simulink model "backstepping_last_good"  (R2023a)
settings: Solver=ode23t  StartTime=0.0  StopTime=inf  RelTol=1e-3
undefined symbols (not defined in the file): K1, K10, K11, K12, K2, K3, K4, K5, K6, K7, K8, K9
libraries: simulink x1, vrlib x1
settings Model: Creator=sait karadeniz  LastModifiedBy=sait karadeniz
settings DataIOCC: ReturnWorkspaceOutputs=off

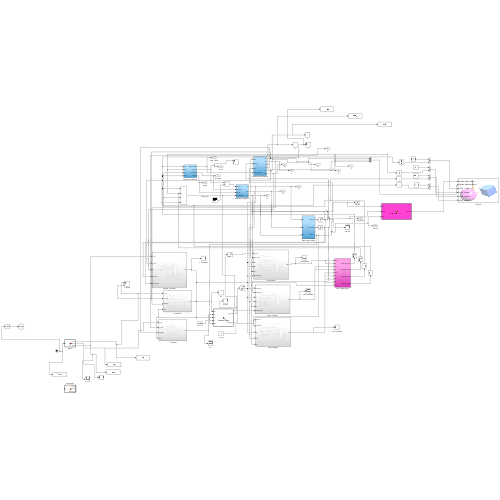
[thumbnail: Simulink's stored preview of the top-level diagram]
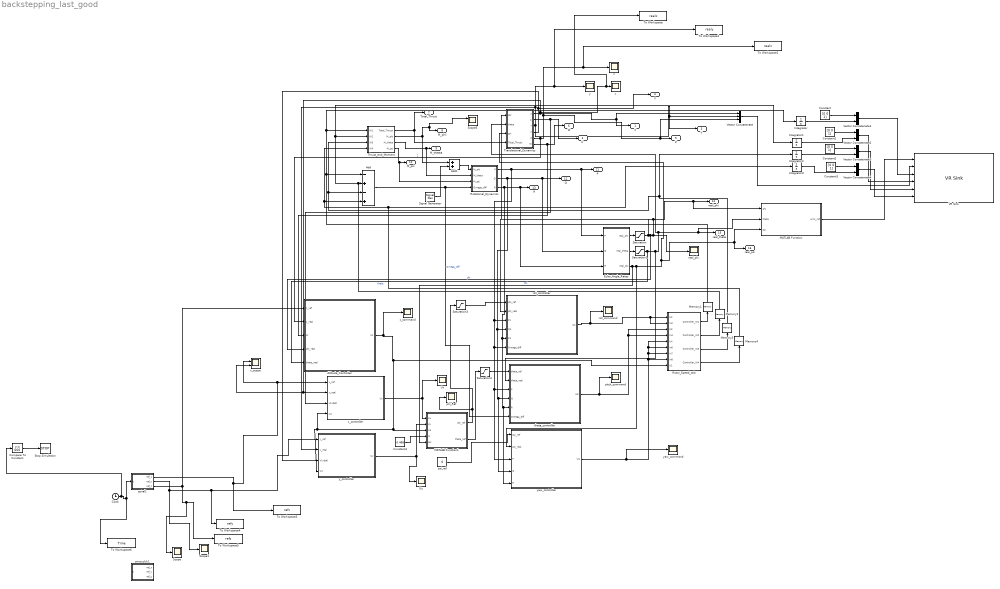
== system backstepping_last_good ==
  Add : Sum  Inputs=-+-+
  Add1 : Sum
  Altitude_Controller : Subsystem
  Clock : Clock
  Compare To Constant : simulink/Logic and Bit Operations/Compare To Constant  relop=>=  const=600  OutDataTypeStr=boolean
  Constant{,1..3} (4 alike) : Constant  Value=[0 0 1]  OutMax=[3]
  Constant4 : Constant  Value=0.468
  Euler_Angle_Rates : Subsystem
  Integrator{,1..3} (4 alike) : Integrator
  MATLAB Function : MATLAB Function  TreatAsAtomicUnit=on
  MATLAB Function1 : MATLAB Function  TreatAsAtomicUnit=on
  Memory{1..4} (4 alike) : Memory
  Rotational_Dynamics : Subsystem
  Rotor_Speed_calc : Subsystem
  Saturation : Saturate  UpperLimit=pi/2  LowerLimit=-pi/2
  Saturation1 : Saturate  UpperLimit=pi/2  LowerLimit=-pi/2
  Saturation2 : Saturate  UpperLimit=0.3  LowerLimit=-0.3
  Saturation3 : Saturate  UpperLimit=0.3  LowerLimit=-0.3
  Scope : Scope
  Scope1 : Scope
  Scope5 : Scope  NumInputPorts=2
  Signal Generator : SignalGenerator  Amplitude=0  Frequency=2  Units=rad/sec
  Stop Simulation : Stop
  Thrust_and_Moment : Subsystem
  To Workspace : ToWorkspace  VariableName=realx  SampleTime=-1
  To Workspace1 : ToWorkspace  VariableName=realy  SampleTime=-1
  To Workspace2 : ToWorkspace  VariableName=realz  SampleTime=-1
  To Workspace3 : ToWorkspace  VariableName=refx  SampleTime=-1
  To Workspace4 : ToWorkspace  VariableName=refy  SampleTime=-1
  To Workspace5 : ToWorkspace  VariableName=refz  SampleTime=-1
  To Workspace6 : ToWorkspace  VariableName=Time  SampleTime=-1
  Translational_Dynamics : Subsystem
  Ux : Scope
  Uy : Scope
  VR Sink : vrlib/VR Sink  InstantiateOnLoad=on  SampleTime=0.1  ViewEnable=on  RemoteChange=off  RemoteView=off  FieldsWritten=DRONE_BODY.rotation.4.1.1.double#DRONE_BODY.translation.3.1.1.double#PROP_1.rotation.4.1.1.double#PROP_2.rotation.4.1.1.double#PROP_3.rotation.4.1.1.double#PROP_4.rotation.4.1.1.double  WorldFileName=C:\Documents\quadcopter.wrl  WorldDescription=Quadcopter World  AutoView=on  VideoDimensions=[]  AllowVariableSize=off
  Vector Concatenate : Concatenate  NumInputs=3
  Vector Concatenate{1..4} (4 alike) : Concatenate
  phi_Ref : Scope
  pitch_command : Scope
  psi_ref : Constant  Value=0
  real_phi. : Scope
  roll_command : Scope
  roll_controller : Subsystem
  sonsuzluk1 : MATLAB Function  TreatAsAtomicUnit=on
  spiral1 : MATLAB Function  TreatAsAtomicUnit=on
  theta_controller : Subsystem
  x : Scope
  x_controller : Subsystem
  x_scope : Scope  NumInputPorts=2
  y : Scope
  y_controller : Subsystem
  yaw_command : Scope
  yaw_controller : Subsystem
  z : Scope
  z_command : Scope
  X : Outport
  U : Outport  Port=2
  Y : Outport  Port=3
  V : Outport  Port=4
  Z : Outport  Port=5
  W : Outport  Port=6
  Total_Thrust : Outport  Port=7
  M_phii : Outport  Port=8
  M_thetaa : Outport  Port=9
  M_psi : Outport  Port=10
  P : Outport  Port=11
  Q : Outport  Port=12
  R : Outport  Port=13
  real_phi : Outport  Port=14
  real_theta : Outport  Port=15
  real_psi : Outport  Port=16
  wires:
  Euler_Angle_Rates/3(real_psi) -> MATLAB Function1/5(psi), yaw_controller/2(psi_real), Translational_Dynamics/3(psi), MATLAB Function/3(psi), real_psi/1  "psi"
  Thrust_and_Moment/2(M_phi) -> Add1/1, M_phii/1, Scope5/1
  Vector Concatenate1/1 -> VR Sink/3
  Rotational_Dynamics/1(P) -> roll_controller/6(Omega_diff), yaw_controller/3(P), theta_controller/3(P), roll_controller/3(P1), P/1, Euler_Angle_Rates/1(P)
  Rotational_Dynamics/2(Q) -> roll_controller/4(Q1), yaw_controller/4(Q), theta_controller/4(Q), Euler_Angle_Rates/2(Q), Q/1
  Integrator/1 -> Vector Concatenate1/2
  Translational_Dynamics/2(U) -> x_controller/3(U(xdot)), U/1
  Saturation1/1 -> Altitude_Controller/5(theta_real), theta_controller/2(theta_real), Translational_Dynamics/2(theta), real_theta/1, MATLAB Function/2(theta)  "theta"
  Vector Concatenate/1 -> VR Sink/2
  Saturation/1 -> roll_controller/2(phi_real), Altitude_Controller/4(phi_real), real_phi./1, Translational_Dynamics/1(phi), MATLAB Function/1(phi), real_phi/1  "phi"
  Thrust_and_Moment/1(Total_Thrust) -> Total_Thrust/1, Translational_Dynamics/4(Total_Thrust)
  Translational_Dynamics/4(V) -> y_controller/3(V(ydot)), V/1
  Euler_Angle_Rates/1(real_phi) -> Saturation/1
  Vector Concatenate2/1 -> VR Sink/4
  Rotor_Speed_calc/2(Controller_W2) -> Memory2/1
  Constant/1 -> Vector Concatenate1/1
  Thrust_and_Moment/4(M_psi) -> Rotational_Dynamics/3(M_psi), M_psi/1
  Rotational_Dynamics/3(R) -> Euler_Angle_Rates/3(R), R/1, roll_controller/5(R1), yaw_controller/5(R), theta_controller/5(R)
  Translational_Dynamics/6(W) -> Altitude_Controller/3(W), W/1
  Integrator1/1 -> Vector Concatenate2/2
  Rotor_Speed_calc/3(Controller_W3) -> Memory3/1
  Vector Concatenate4/1 -> VR Sink/6
  Integrator3/1 -> Vector Concatenate4/2
  MATLAB Function/1(vrml_rot) -> VR Sink/1
  Translational_Dynamics/5(Z) -> Altitude_Controller/2(z_real), To Workspace2/1, z/1, Z/1, Vector Concatenate/3  "Z"
  Thrust_and_Moment/3(M_theta) -> M_thetaa/1, Rotational_Dynamics/2(M_theta)
  Rotor_Speed_calc/1(Controller_W1) -> Memory1/1
  Rotor_Speed_calc/4(Controller_W4) -> Memory4/1
  Constant3/1 -> Vector Concatenate4/1
  Vector Concatenate3/1 -> VR Sink/5
  Constant2/1 -> Vector Concatenate3/1
  Euler_Angle_Rates/2(real_theta) -> Saturation1/1
  Add/1 -> theta_controller/6(Omega_diff), Rotational_Dynamics/4(Omega_diff)  "Omega_diff"
  Constant1/1 -> Vector Concatenate2/1
  Integrator2/1 -> Vector Concatenate3/2
  spiral1/1(ref_x) -> x_controller/1(x_ref), x_scope/1, To Workspace3/1
  MATLAB Function1/1(phi_ref) -> Saturation3/1, phi_Ref/1
  MATLAB Function1/2(theta_ref) -> Saturation2/1
  psi_ref/1 -> yaw_controller/1(psi_ref)
  spiral1/2(ref_y) -> Scope1/1, y_controller/1(y_ref), To Workspace4/1
  spiral1/3(ref_z) -> Scope/1, To Workspace5/1, Altitude_Controller/1(z_ref)
  roll_controller/1(U2) -> roll_command/1, Rotor_Speed_calc/2(In2), Rotor_Speed_calc/1(U2)
  theta_controller/1(U3) -> pitch_command/1, Rotor_Speed_calc/4(In4), Rotor_Speed_calc/3(U3)
  yaw_controller/1(U4) -> yaw_command/1, Rotor_Speed_calc/8(In8), Rotor_Speed_calc/7(In7), Rotor_Speed_calc/6(In6), Rotor_Speed_calc/5(U4)
  x_controller/1(Ux) -> MATLAB Function1/1(Ux), Ux/1
  y_controller/1(Uy) -> MATLAB Function1/2(Uy), Uy/1
  Memory1/1 -> Integrator/1, Thrust_and_Moment/1(W1), Add/1
  Memory2/1 -> Integrator1/1, Thrust_and_Moment/2(W2), Add/2
  Memory3/1 -> Integrator2/1, Thrust_and_Moment/3(W3), Add/3
  Memory4/1 -> Thrust_and_Moment/4(W4), Add/4, Integrator3/1
  Saturation2/1 -> theta_controller/1(theta_ref)
  Constant4/1 -> MATLAB Function1/4(m)
  Altitude_Controller/1(U1) -> Rotor_Speed_calc/9(U1), MATLAB Function1/3(U1), y_controller/4(U1), x_controller/4(U1), z_command/1
  Saturation3/1 -> roll_controller/1(phi_ref)
  Signal Generator/1 -> Add1/2
  Add1/1 -> Rotational_Dynamics/1(M_phi)
  Compare To Constant/1 -> Stop Simulation/1
  Clock/1 -> Compare To Constant/1, spiral1/1(t), To Workspace6/1
  Translational_Dynamics/3(Y) -> y_controller/2(y_real), To Workspace1/1, y/1, Y/1, Vector Concatenate/2
  Translational_Dynamics/1(X) -> x_controller/2(x_real), x_scope/2, To Workspace/1, x/1, Vector Concatenate/1, X/1

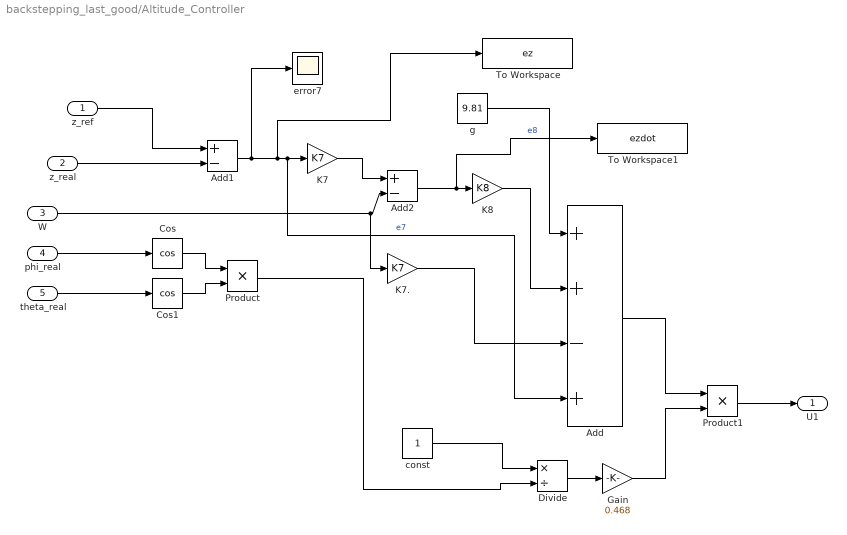
== system backstepping_last_good/Altitude_Controller ==
  z_ref : Inport
  z_real : Inport  Port=2
  W : Inport  Port=3
  phi_real : Inport  Port=4
  theta_real : Inport  Port=5
  Add : Sum  Inputs=++-+
  Add1 : Sum  Inputs=+-
  Add2 : Sum  Inputs=+-
  Cos : Trigonometry  Operator=cos
  Cos1 : Trigonometry  Operator=cos
  Divide : Product  Inputs=*/
  Gain : Gain  Gain=0.468
  K7 : Gain  Gain=K7
  K7. : Gain  Gain=K7
  K8 : Gain  Gain=K8
  Product : Product
  Product1 : Product
  To Workspace : ToWorkspace  VariableName=ez  SampleTime=-1
  To Workspace1 : ToWorkspace  VariableName=ezdot  SampleTime=-1
  const : Constant
  error7 : Scope
  g : Constant  Value=9.81
  U1 : Outport
  wires:
  z_ref/1 -> Add1/1
  Add1/1 -> error7/1, To Workspace/1, Add/4, K7/1  "e7"
  K7/1 -> Add2/1
  W/1 -> Add2/2, K7./1
  Add2/1 -> To Workspace1/1, K8/1  "e8"
  phi_real/1 -> Cos/1
  theta_real/1 -> Cos1/1
  Cos/1 -> Product/1
  Cos1/1 -> Product/2
  Product/1 -> Divide/2
  const/1 -> Divide/1
  K8/1 -> Add/2
  g/1 -> Add/1
  K7./1 -> Add/3
  Add/1 -> Product1/1
  Divide/1 -> Gain/1
  Product1/1 -> U1/1
  z_real/1 -> Add1/2
  Gain/1 -> Product1/2

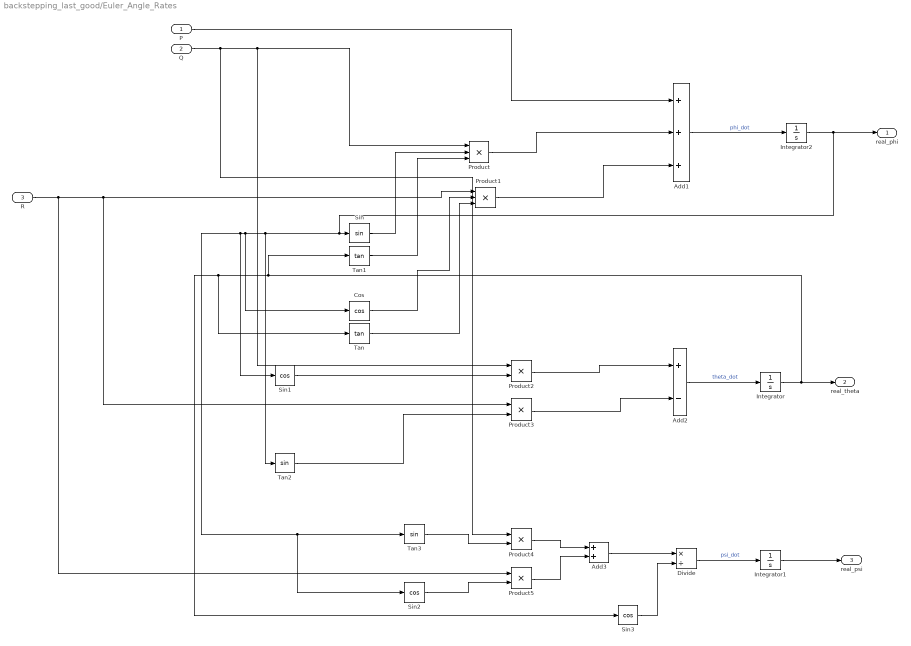
== system backstepping_last_good/Euler_Angle_Rates ==
  P : Inport
  Q : Inport  Port=2
  R : Inport  Port=3
  Add1 : Sum  Inputs=+++
  Add2 : Sum  Inputs=+-
  Add3 : Sum
  Cos : Trigonometry  Operator=cos
  Divide : Product  Inputs=*/
  Integrator : Integrator
  Integrator1 : Integrator
  Integrator2 : Integrator
  Product : Product  Inputs=3
  Product1 : Product  Inputs=3
  Product{2..5} (4 alike) : Product
  Sin : Trigonometry
  Sin1 : Trigonometry  Operator=cos
  Sin2 : Trigonometry  Operator=cos
  Sin3 : Trigonometry  Operator=cos
  Tan : Trigonometry  Operator=tan
  Tan1 : Trigonometry  Operator=tan
  Tan2 : Trigonometry
  Tan3 : Trigonometry
  real_phi : Outport
  real_theta : Outport  Port=2
  real_psi : Outport  Port=3
  wires:
  Tan1/1 -> Product/3
  Integrator2/1 -> real_phi/1, Sin2/1, Tan3/1, Sin1/1, Cos/1, Tan2/1, Sin/1
  Add1/1 -> Integrator2/1  "phi_dot"
  Divide/1 -> Integrator1/1  "psi_dot"
  Product3/1 -> Add2/2
  Integrator/1 -> real_theta/1, Sin3/1, Tan/1, Tan1/1
  Product1/1 -> Add1/3
  Tan3/1 -> Product4/2
  Sin2/1 -> Product5/2
  Tan2/1 -> Product3/2
  Integrator1/1 -> real_psi/1
  Product2/1 -> Add2/1
  Cos/1 -> Product1/2
  Add2/1 -> Integrator/1  "theta_dot"
  Product4/1 -> Add3/1
  Sin/1 -> Product/2
  Tan/1 -> Product1/3
  Add3/1 -> Divide/1
  Product/1 -> Add1/2
  Sin1/1 -> Product2/2
  Product5/1 -> Add3/2
  Sin3/1 -> Divide/2
  Q/1 -> Product4/1, Product/1, Product2/1
  R/1 -> Product5/1, Product3/1, Product1/1
  P/1 -> Add1/1

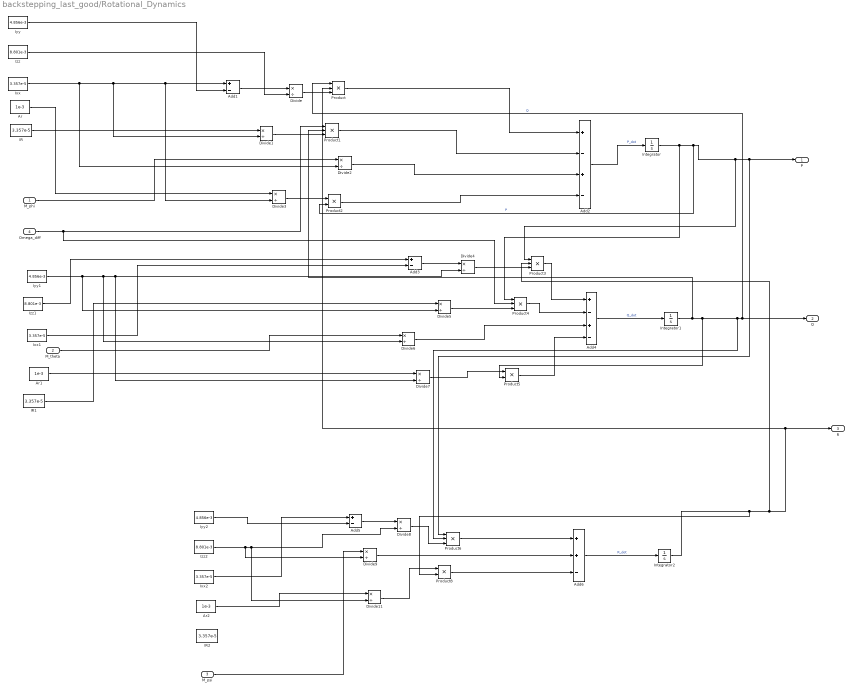
== system backstepping_last_good/Rotational_Dynamics ==
  M_phi : Inport
  M_theta : Inport  Port=2
  M_psi : Inport  Port=3
  Omega_diff : Inport  Port=4
  Add1 : Sum  Inputs=+-
  Add2 : Sum  Inputs=+-+-
  Add3 : Sum  Inputs=+-
  Add4 : Sum  Inputs=+-+-
  Add5 : Sum  Inputs=+-
  Add6 : Sum  Inputs=++-
  Ar : Constant  Value=1e-3
  Ar1 : Constant  Value=1e-3
  Ar2 : Constant  Value=1e-3
  Divide{,1..9,11} (11 alike) : Product  Inputs=*/
  IR : Constant  Value=3.357e-5
  IR1 : Constant  Value=3.357e-5
  IR2 : Constant  Value=3.357e-5
  Integrator : Integrator
  Integrator1 : Integrator
  Integrator2 : Integrator
  Ixx : Constant  Value=3.357e-5
  Ixx1 : Constant  Value=3.357e-5
  Ixx2 : Constant  Value=3.357e-5
  Iyy : Constant  Value=4.856e-3
  Iyy1 : Constant  Value=4.856e-3
  Iyy2 : Constant  Value=4.856e-3
  Izz : Constant  Value=8.801e-3
  Izz1 : Constant  Value=8.801e-3
  Izz2 : Constant  Value=8.801e-3
  Product{,1,3..4,6} (5 alike) : Product  Inputs=3
  Product2 : Product
  Product5 : Product
  Product8 : Product
  P : Outport
  Q : Outport  Port=2
  R : Outport  Port=3
  wires:
  Integrator/1 -> Product4/1, Product2/2, Product3/1, Product6/1, P/1  "P"
  Product6/1 -> Add6/1
  Add6/1 -> Integrator2/1  "R_dot"
  Divide2/1 -> Add2/3
  Add3/1 -> Divide4/1
  Add5/1 -> Divide8/1
  Divide3/1 -> Product2/1
  Integrator1/1 -> Product1/2, Product5/2, Product/1, Q/1, Product6/2  "Q"
  Product/1 -> Add2/1
  Product1/1 -> Add2/2
  Divide11/1 -> Product8/1
  Add1/1 -> Divide/1
  Product5/1 -> Add4/4
  Integrator2/1 -> Product8/2, Product3/2, R/1, Product/2
  Divide8/1 -> Product6/3
  Product3/1 -> Add4/1
  Add2/1 -> Integrator/1  "P_dot"
  Product2/1 -> Add2/4
  Divide5/1 -> Product4/3
  Divide4/1 -> Product3/3
  Divide6/1 -> Add4/3
  Divide7/1 -> Product5/1
  Product4/1 -> Add4/2
  Add4/1 -> Integrator1/1  "Q_dot"
  Divide9/1 -> Add6/2
  Divide/1 -> Product/3
  Divide1/1 -> Product1/3
  Product8/1 -> Add6/3
  Ixx/1 -> Divide2/2, Divide1/2, Divide3/2, Add1/1
  IR/1 -> Divide1/1
  Omega_diff/1 -> Product4/2, Product1/1
  M_phi/1 -> Divide2/1
  Ar/1 -> Divide3/1
  Iyy/1 -> Add1/2
  Izz/1 -> Divide/2
  Izz1/1 -> Add3/1
  Ixx1/1 -> Add3/2
  Iyy1/1 -> Divide5/2, Divide6/2, Divide7/2, Divide4/2
  IR1/1 -> Divide5/1
  M_theta/1 -> Divide6/1
  Ar1/1 -> Divide7/1
  Ixx2/1 -> Add5/1
  Iyy2/1 -> Add5/2
  Izz2/1 -> Divide9/2, Divide11/2, Divide8/2
  M_psi/1 -> Divide9/1
  Ar2/1 -> Divide11/1

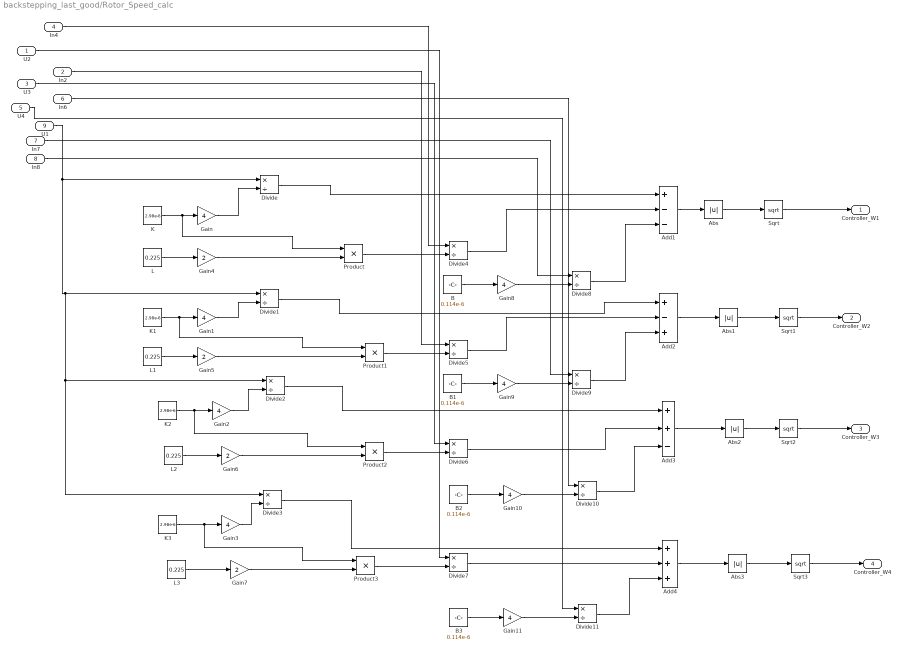
== system backstepping_last_good/Rotor_Speed_calc ==
  U2 : Inport
  In2 : Inport  Port=2
  U3 : Inport  Port=3
  In4 : Inport  Port=4
  U4 : Inport  Port=5
  In6 : Inport  Port=6
  In7 : Inport  Port=7
  In8 : Inport  Port=8
  U1 : Inport  Port=9
  Abs{,1..3} (4 alike) : Abs  SaturateOnIntegerOverflow=off
  Add1 : Sum  Inputs=+--
  Add2 : Sum  Inputs=+-+
  Add3 : Sum  Inputs=++-
  Add4 : Sum  Inputs=+++
  B{,1..3} (4 alike) : Constant  Value=0.114e-6
  Divide{,1..11} (12 alike) : Product  Inputs=*/
  Gain{,1..3,8..11} (8 alike) : Gain  Gain=4
  Gain{4..7} (4 alike) : Gain  Gain=2
  K{,1..3} (4 alike) : Constant  Value=2.98e-6
  L{,1..3} (4 alike) : Constant  Value=0.225
  Product{,1..3} (4 alike) : Product
  Sqrt{,1..3} (4 alike) : Sqrt
  Controller_W1 : Outport
  Controller_W2 : Outport  Port=2
  Controller_W3 : Outport  Port=3
  Controller_W4 : Outport  Port=4
  wires:
  K/1 -> Product/1, Gain/1
  Sqrt1/1 -> Controller_W2/1
  Divide1/1 -> Add2/1
  Divide/1 -> Add1/1
  Gain3/1 -> Divide3/2
  Gain/1 -> Divide/2
  Divide8/1 -> Add1/3
  Add4/1 -> Abs3/1
  B/1 -> Gain8/1
  B2/1 -> Gain10/1
  Gain5/1 -> Product1/2
  Divide9/1 -> Add2/3
  Abs2/1 -> Sqrt2/1
  Add2/1 -> Abs1/1
  Divide5/1 -> Add2/2
  B3/1 -> Gain11/1
  Add3/1 -> Abs2/1
  Divide11/1 -> Add4/3
  Divide10/1 -> Add3/3
  K1/1 -> Product1/1, Gain1/1
  Divide4/1 -> Add1/2
  U1/1 -> Divide3/1, Divide2/1, Divide1/1, Divide/1
  Product3/1 -> Divide7/2
  Product/1 -> Divide4/2
  K2/1 -> Product2/1, Gain2/1
  Divide2/1 -> Add3/1
  Gain1/1 -> Divide1/2
  Divide3/1 -> Add4/1
  Divide7/1 -> Add4/2
  L1/1 -> Gain5/1
  Gain9/1 -> Divide9/2
  Abs3/1 -> Sqrt3/1
  L/1 -> Gain4/1
  Abs1/1 -> Sqrt1/1
  B1/1 -> Gain9/1
  Sqrt/1 -> Controller_W1/1
  Gain4/1 -> Product/2
  L2/1 -> Gain6/1
  In8/1 -> Divide8/1
  U4/1 -> Divide11/1
  Gain6/1 -> Product2/2
  U3/1 -> Divide6/1
  Product1/1 -> Divide5/2
  Product2/1 -> Divide6/2
  U2/1 -> Divide7/1
  Divide6/1 -> Add3/2
  Gain8/1 -> Divide8/2
  L3/1 -> Gain7/1
  Sqrt3/1 -> Controller_W4/1
  K3/1 -> Product3/1, Gain3/1
  Gain10/1 -> Divide10/2
  Gain7/1 -> Product3/2
  Gain11/1 -> Divide11/2
  Gain2/1 -> Divide2/2
  Sqrt2/1 -> Controller_W3/1
  Abs/1 -> Sqrt/1
  Add1/1 -> Abs/1
  In4/1 -> Divide4/1
  In6/1 -> Divide10/1
  In7/1 -> Divide9/1
  In2/1 -> Divide5/1

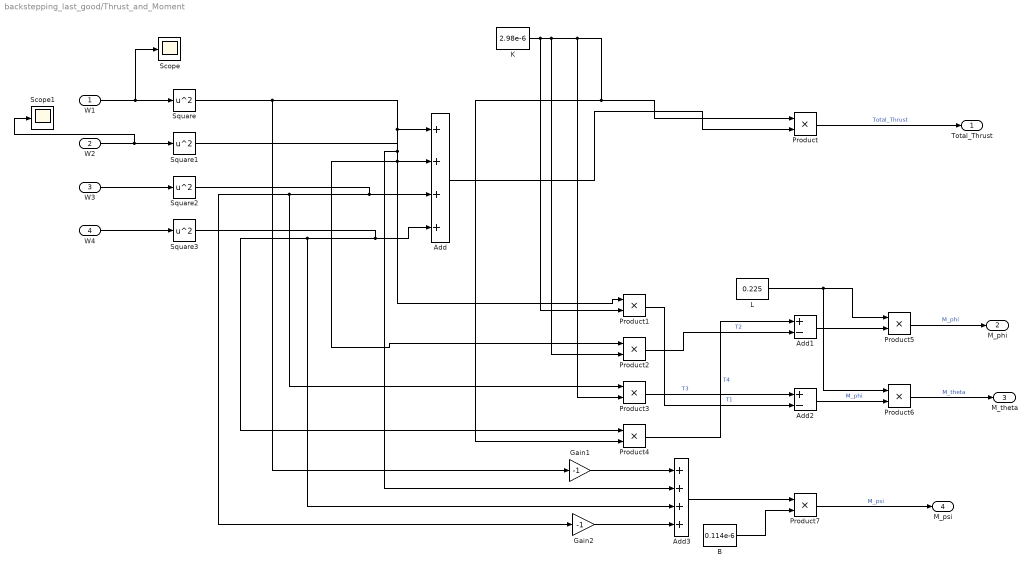
== system backstepping_last_good/Thrust_and_Moment ==
  W1 : Inport
  W2 : Inport  Port=2
  W3 : Inport  Port=3
  W4 : Inport  Port=4
  Add : Sum  Inputs=++++
  Add1 : Sum  Inputs=+-
  Add2 : Sum  Inputs=+-
  Add3 : Sum  Inputs=++++
  B : Constant  Value=0.114e-6
  Gain1 : Gain  Gain=-1
  Gain2 : Gain  Gain=-1
  K : Constant  Value=2.98e-6
  L : Constant  Value=0.225
  Product{,1..7} (8 alike) : Product
  Scope : Scope
  Scope1 : Scope
  Square{,1..3} (4 alike) : Math  Operator=square
  Total_Thrust : Outport
  M_phi : Outport  Port=2
  M_theta : Outport  Port=3
  M_psi : Outport  Port=4
  wires:
  Square1/1 -> Add3/2, Add/2, Product2/1
  Product3/1 -> Add2/1  "T3"
  Product1/1 -> Add2/2  "T1"
  Square3/1 -> Product4/1, Add3/3, Add/4
  Add3/1 -> Product7/1
  Square2/1 -> Gain2/1, Product3/1, Add/3
  Product7/1 -> M_psi/1  "M_psi"
  W1/1 -> Scope/1, Square/1
  K/1 -> Product2/2, Product4/2, Product/1, Product3/2, Product1/2
  W4/1 -> Square3/1
  Product2/1 -> Add1/2  "T2"
  Add1/1 -> Product5/2
  W2/1 -> Scope1/1, Square1/1
  Product5/1 -> M_phi/1  "M_phi"
  Square/1 -> Add/1, Product1/1, Gain1/1
  Product/1 -> Total_Thrust/1  "Total_Thrust"
  Gain2/1 -> Add3/4
  L/1 -> Product6/1, Product5/1
  Add2/1 -> Product6/2  "M_phi"
  W3/1 -> Square2/1
  B/1 -> Product7/2
  Product4/1 -> Add1/1  "T4"
  Add/1 -> Product/2
  Gain1/1 -> Add3/1
  Product6/1 -> M_theta/1  "M_theta"

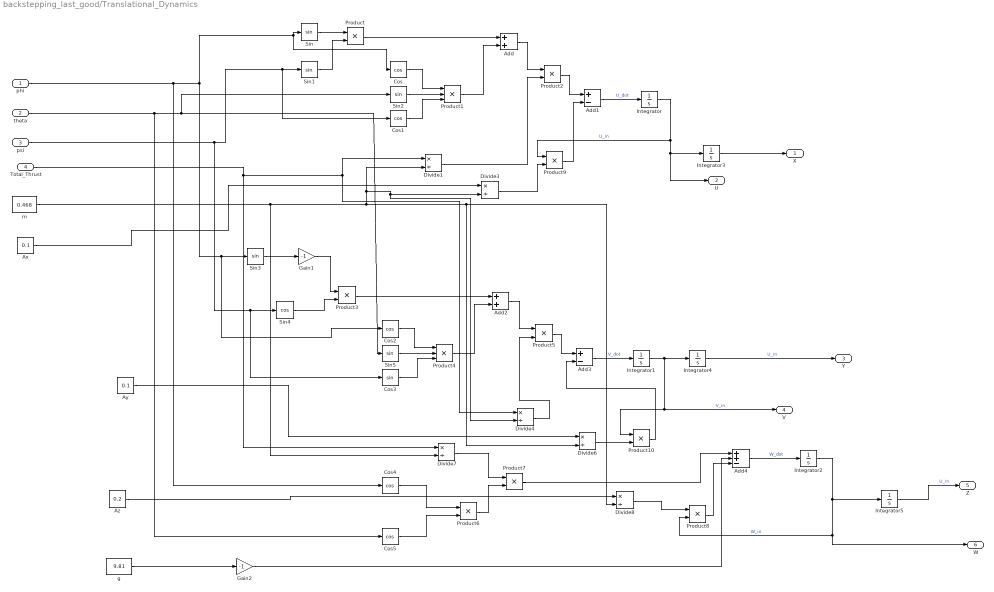
== system backstepping_last_good/Translational_Dynamics ==
  phi : Inport
  theta : Inport  Port=2
  psi : Inport  Port=3
  Total_Thrust : Inport  Port=4
  Add : Sum
  Add1 : Sum  Inputs=+-
  Add2 : Sum
  Add3 : Sum  Inputs=+-
  Add4 : Sum  Inputs=++-
  Ax : Constant  Value=0.1
  Ay : Constant  Value=0.1
  Az : Constant  Value=0.2
  Cos{,1..2,4..5} (5 alike) : Trigonometry  Operator=cos
  Cos3 : Trigonometry
  Divide{1,3..4,6..8} (6 alike) : Product  Inputs=*/
  Gain1 : Gain  Gain=-1
  Gain2 : Gain  Gain=-1
  Integrator{,1..5} (6 alike) : Integrator
  Product{,2..3,5..10} (9 alike) : Product
  Product1 : Product  Inputs=3
  Product4 : Product  Inputs=3
  Sin{,1..3,5} (5 alike) : Trigonometry
  Sin4 : Trigonometry  Operator=cos
  g : Constant  Value=9.81
  m : Constant  Value=0.468
  X : Outport
  U : Outport  Port=2
  Y : Outport  Port=3
  V : Outport  Port=4
  Z : Outport  Port=5
  W : Outport  Port=6
  wires:
  Integrator1/1 -> Product10/1, V/1, Integrator4/1  "V_in"
  m/1 -> Divide7/2, Divide8/2, Divide6/2, Divide3/2, Divide4/2, Divide1/2
  Integrator2/1 -> Integrator5/1, W/1, Product8/2  "W_in"
  Product8/1 -> Add4/3
  Ay/1 -> Divide6/1
  Product2/1 -> Add1/1
  Integrator/1 -> Product9/1, U/1, Integrator3/1  "U_in"
  g/1 -> Gain2/1
  Product6/1 -> Product7/2
  phi/1 -> Cos2/1, Sin3/1, Sin/1, Cos/1, Cos4/1
  Integrator3/1 -> X/1
  Integrator5/1 -> Z/1  "U_in"
  Product7/1 -> Add4/1
  psi/1 -> Cos3/1, Sin4/1, Cos1/1, Sin1/1
  Product4/1 -> Add2/2
  Divide1/1 -> Product2/2
  Product9/1 -> Add1/2
  Divide7/1 -> Product7/1
  Sin/1 -> Product/1
  theta/1 -> Sin5/1, Sin2/1, Cos5/1
  Gain2/1 -> Add4/2
  Integrator4/1 -> Y/1  "U_in"
  Add/1 -> Product2/1
  Product1/1 -> Add/2
  Cos4/1 -> Product6/1
  Sin2/1 -> Product1/2
  Add1/1 -> Integrator/1  "U_dot"
  Total_Thrust/1 -> Divide7/1, Divide1/1, Divide4/1
  Cos/1 -> Product1/1
  Add3/1 -> Integrator1/1  "V_dot"
  Gain1/1 -> Product3/1
  Sin1/1 -> Product/2
  Add4/1 -> Integrator2/1  "W_dot"
  Cos5/1 -> Product6/2
  Product/1 -> Add/1
  Divide8/1 -> Product8/1
  Az/1 -> Divide8/1
  Divide3/1 -> Product9/2
  Sin5/1 -> Product4/2
  Cos1/1 -> Product1/3
  Ax/1 -> Divide3/1
  Cos3/1 -> Product4/3
  Product10/1 -> Add3/2
  Divide4/1 -> Product5/2
  Add2/1 -> Product5/1
  Sin4/1 -> Product3/2
  Sin3/1 -> Gain1/1
  Divide6/1 -> Product10/2
  Cos2/1 -> Product4/1
  Product3/1 -> Add2/1
  Product5/1 -> Add3/1

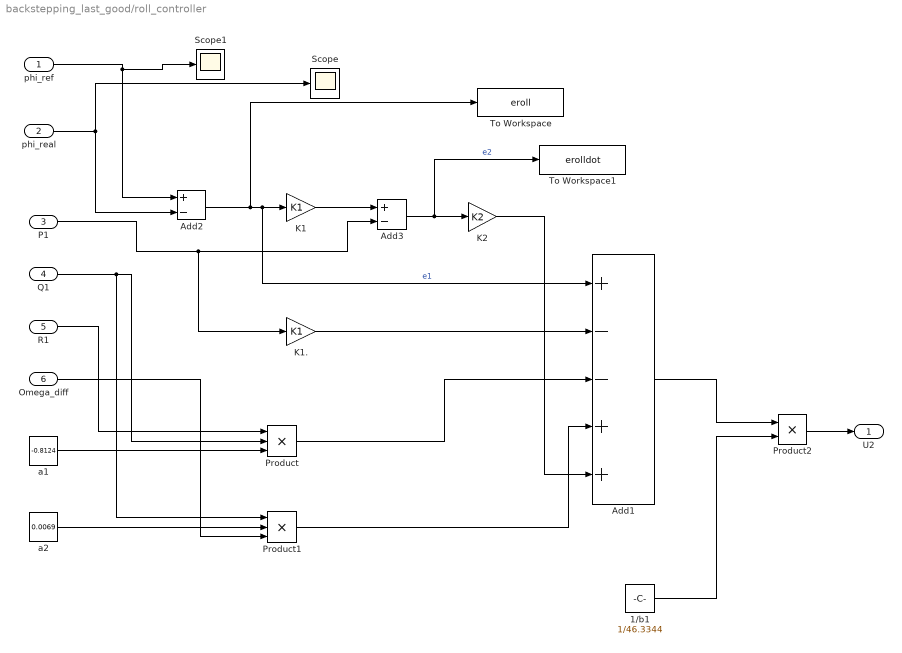
== system backstepping_last_good/roll_controller ==
  phi_ref : Inport
  phi_real : Inport  Port=2
  P1 : Inport  Port=3
  Q1 : Inport  Port=4
  R1 : Inport  Port=5
  Omega_diff : Inport  Port=6
  1/b1 : Constant  Value=1/46.3344
  Add1 : Sum  Inputs=+--++
  Add2 : Sum  Inputs=+-
  Add3 : Sum  Inputs=+-
  K1 : Gain  Gain=K1
  K1. : Gain  Gain=K1
  K2 : Gain  Gain=K2
  Product : Product  Inputs=3
  Product1 : Product  Inputs=3
  Product2 : Product
  Scope : Scope
  Scope1 : Scope
  To Workspace : ToWorkspace  VariableName=eroll  SampleTime=-1
  To Workspace1 : ToWorkspace  VariableName=erolldot  SampleTime=-1
  a1 : Constant  Value=-0.8124
  a2 : Constant  Value=0.0069
  U2 : Outport
  wires:
  1/b1/1 -> Product2/2
  Add1/1 -> Product2/1
  Product2/1 -> U2/1
  P1/1 -> K1./1, Add3/2
  phi_real/1 -> Add2/2, Scope/1
  Q1/1 -> Product1/1, Product/2
  Add3/1 -> To Workspace1/1, K2/1  "e2"
  a2/1 -> Product1/2
  phi_ref/1 -> Scope1/1, Add2/1
  K1/1 -> Add3/1
  K1./1 -> Add1/2
  Product1/1 -> Add1/4
  a1/1 -> Product/3
  R1/1 -> Product/1
  Omega_diff/1 -> Product1/3
  K2/1 -> Add1/5
  Add2/1 -> To Workspace/1, Add1/1, K1/1  "e1"
  Product/1 -> Add1/3

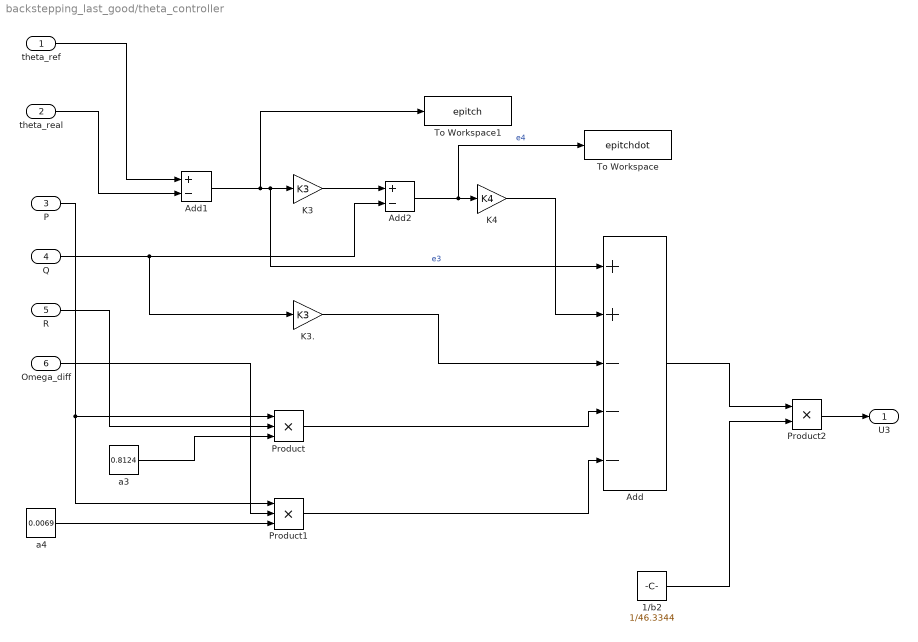
== system backstepping_last_good/theta_controller ==
  theta_ref : Inport
  theta_real : Inport  Port=2
  P : Inport  Port=3
  Q : Inport  Port=4
  R : Inport  Port=5
  Omega_diff : Inport  Port=6
  1/b2 : Constant  Value=1/46.3344
  Add : Sum  Inputs=++---
  Add1 : Sum  Inputs=+-
  Add2 : Sum  Inputs=+-
  K3 : Gain  Gain=K3
  K3. : Gain  Gain=K3
  K4 : Gain  Gain=K4
  Product : Product  Inputs=3
  Product1 : Product  Inputs=3
  Product2 : Product
  To Workspace : ToWorkspace  VariableName=epitchdot  SampleTime=-1
  To Workspace1 : ToWorkspace  VariableName=epitch  SampleTime=-1
  a3 : Constant  Value=0.8124
  a4 : Constant  Value=0.0069
  U3 : Outport
  wires:
  Product2/1 -> U3/1
  1/b2/1 -> Product2/2
  Add/1 -> Product2/1
  Add2/1 -> To Workspace/1, K4/1  "e4"
  K3/1 -> Add2/1
  Add1/1 -> To Workspace1/1, Add/1, K3/1  "e3"
  theta_real/1 -> Add1/2
  theta_ref/1 -> Add1/1
  K4/1 -> Add/2
  Q/1 -> K3./1, Add2/2
  K3./1 -> Add/3
  a3/1 -> Product/3
  R/1 -> Product/2
  P/1 -> Product1/1, Product/1
  Product/1 -> Add/4
  Product1/1 -> Add/5
  a4/1 -> Product1/3
  Omega_diff/1 -> Product1/2

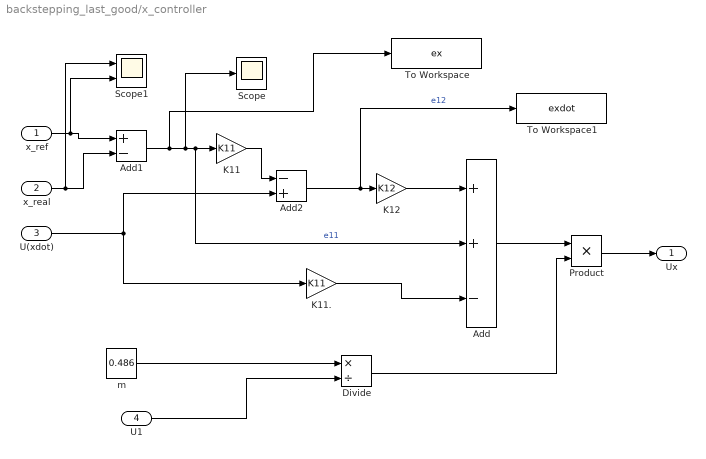
== system backstepping_last_good/x_controller ==
  x_ref : Inport
  x_real : Inport  Port=2
  U(xdot) : Inport  Port=3
  U1 : Inport  Port=4
  Add : Sum  Inputs=++-
  Add1 : Sum  Inputs=+-
  Add2 : Sum  Inputs=-+
  Divide : Product  Inputs=*/
  K11 : Gain  Gain=K11
  K11. : Gain  Gain=K11
  K12 : Gain  Gain=K12
  Product : Product
  Scope : Scope
  Scope1 : Scope  NumInputPorts=2
  To Workspace : ToWorkspace  VariableName=ex  SampleTime=-1
  To Workspace1 : ToWorkspace  VariableName=exdot  SampleTime=-1
  m : Constant  Value=0.486
  Ux : Outport
  wires:
  x_ref/1 -> Scope1/2, Add1/1
  x_real/1 -> Scope1/1, Add1/2
  Add1/1 -> To Workspace/1, Scope/1, Add/2, K11/1  "e11"
  K11/1 -> Add2/1
  Add2/1 -> To Workspace1/1, K12/1  "e12"
  K12/1 -> Add/1
  K11./1 -> Add/3
  m/1 -> Divide/1
  U1/1 -> Divide/2
  Add/1 -> Product/1
  Divide/1 -> Product/2
  Product/1 -> Ux/1
  U(xdot)/1 -> K11./1, Add2/2

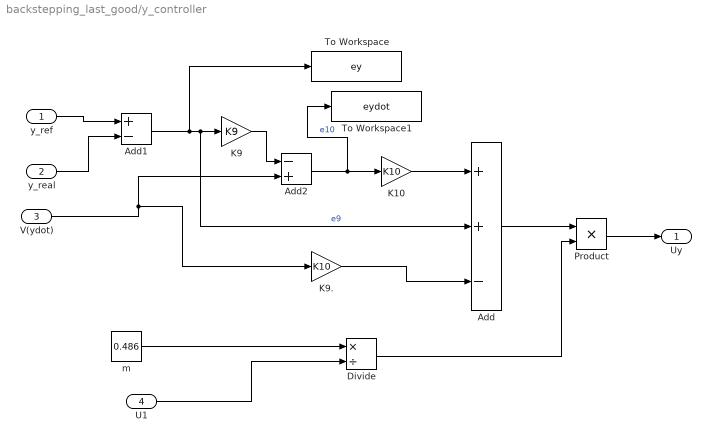
== system backstepping_last_good/y_controller ==
  y_ref : Inport
  y_real : Inport  Port=2
  V(ydot) : Inport  Port=3
  U1 : Inport  Port=4
  Add : Sum  Inputs=++-
  Add1 : Sum  Inputs=+-
  Add2 : Sum  Inputs=-+
  Divide : Product  Inputs=*/
  K10 : Gain  Gain=K10
  K9 : Gain  Gain=K9
  K9. : Gain  Gain=K10
  Product : Product
  To Workspace : ToWorkspace  VariableName=ey  SampleTime=-1
  To Workspace1 : ToWorkspace  VariableName=eydot  SampleTime=-1
  m : Constant  Value=0.486
  Uy : Outport
  wires:
  Product/1 -> Uy/1
  Divide/1 -> Product/2
  Add/1 -> Product/1
  U1/1 -> Divide/2
  m/1 -> Divide/1
  K9./1 -> Add/3
  K10/1 -> Add/1
  Add2/1 -> To Workspace1/1, K10/1  "e10"
  K9/1 -> Add2/1
  V(ydot)/1 -> K9./1, Add2/2
  Add1/1 -> To Workspace/1, K9/1, Add/2  "e9"
  y_real/1 -> Add1/2
  y_ref/1 -> Add1/1

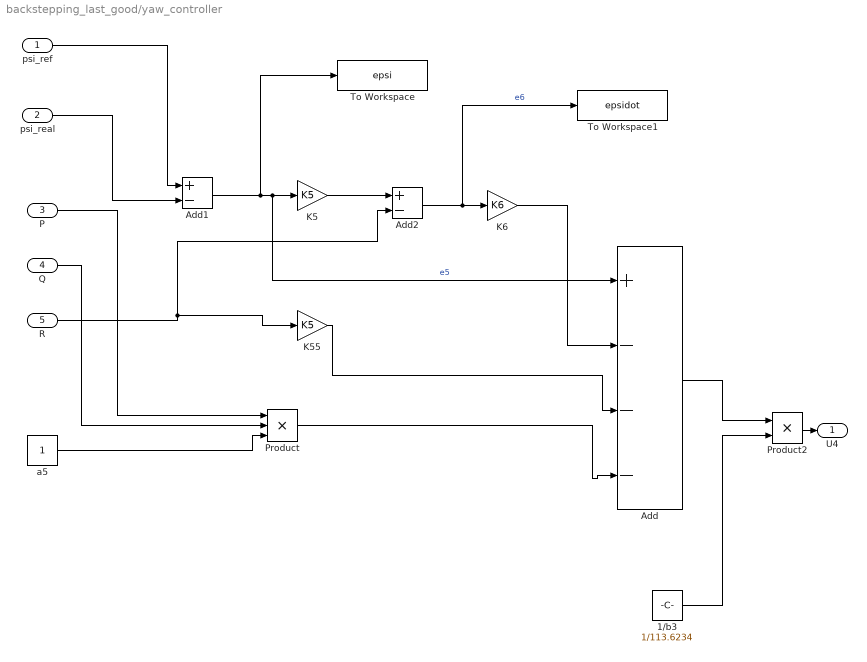
== system backstepping_last_good/yaw_controller ==
  psi_ref : Inport
  psi_real : Inport  Port=2
  P : Inport  Port=3
  Q : Inport  Port=4
  R : Inport  Port=5
  1/b3 : Constant  Value=1/113.6234
  Add : Sum  Inputs=+---
  Add1 : Sum  Inputs=+-
  Add2 : Sum  Inputs=+-
  K5 : Gain  Gain=K5
  K55 : Gain  Gain=K5
  K6 : Gain  Gain=K6
  Product : Product  Inputs=3
  Product2 : Product
  To Workspace : ToWorkspace  VariableName=epsi  SampleTime=-1
  To Workspace1 : ToWorkspace  VariableName=epsidot  SampleTime=-1
  a5 : Constant
  U4 : Outport
  wires:
  Add1/1 -> To Workspace/1, Add/1, K5/1  "e5"
  K5/1 -> Add2/1
  Add2/1 -> To Workspace1/1, K6/1  "e6"
  Add/1 -> Product2/1
  1/b3/1 -> Product2/2
  Product2/1 -> U4/1
  psi_ref/1 -> Add1/1
  psi_real/1 -> Add1/2
  R/1 -> K55/1, Add2/2
  K6/1 -> Add/2
  K55/1 -> Add/3
  P/1 -> Product/1
  Q/1 -> Product/2
  a5/1 -> Product/3
  Product/1 -> Add/4

== matlab function backstepping_last_good/MATLAB Function1 ==
  data: Ux input; phi_ref output; Uy input; U1 input; m input; psi input; theta_ref output
function [phi_ref, theta_ref] = Inversion_Block(Ux, Uy, U1, m, psi)
% Ux, Uy: X/Y Kontrolcülerinden gelen sanal ivme komutları
% U1: Z Kontrolcüsünden gelen toplam itki komutu
% m: Kütle
% psi: Gerçek Yaw Açısı

    %% Güvenlik Limiti
    limit = 0.98; 
    
    % U1'in sıfıra yaklaşmasını önle
    if U1 < 0.1
        U1 = 0.1; 
    end

    %% 1. Phi_ref (Roll) Hesabı
    
    % Doğru Formülün Pay Kısmı:
    numerator_phi = m * (Ux * sin(psi) - Uy * cos(psi));
    
    % Payda (U1):
    denominator_phi = U1;
    
    term_phi = numerator_phi / denominator_phi;
    
    % Sinyal Sınırlama (Saturation)
    if term_phi > limit
        term_phi = limit;
    elseif term_phi < -limit
        term_phi = -limit;
    end
    
    phi_ref = asin(term_phi);

    %% 2. Theta_ref (Pitch) Hesabı

    % Doğru Formülün Pay Kısmı:
    numerator_theta = m * (Ux * cos(psi) + Uy * sin(psi));
    
    % Payda:
    denominator_theta = U1 * cos(phi_ref);
    
    % Payda sıfıra çok yaklaşırsa bölme hatası olmasın
    if abs(denominator_theta) < 0.05
        denominator_theta = 0.05; 
    end
    
    term_theta = numerator_theta / denominator_theta;
    
    % Sinyal Sınırlama (Saturation)
    if term_theta > limit
        term_theta = limit;
    elseif term_theta < -limit
        term_theta = -limit;
    end
    
    theta_ref = asin(term_theta);

end

== matlab function backstepping_last_good/MATLAB Function ==
  data: phi input; vrml_rot output; theta input; psi input
function vrml_rot = EulerToVRMLRot(phi, theta, psi)
% Bu fonksiyon, roll (phi), pitch (theta) ve yaw (psi) Euler açılarını
% VRML'nin beklediği Axis-Angle formatına dönüştürür.
% Girişler (radyan cinsinden):
% phi   : Roll açısı (X ekseni etrafında)
% theta : Pitch açısı (Y ekseni etrafında)
% psi   : Yaw açısı (Z ekseni etrafında)
% Çıkış (Axis-Angle formatında):
% vrml_rot = [eksen_x, eksen_y, eksen_z, açı_radyan]

% Genellikle MATLAB ve VRML arasındaki koordinat sistemi farklarını
% ve Euler açı sıra konvansiyonunu dikkate almak gerekir.
% Burada Z-Y-X (Yaw-Pitch-Roll) Euler dönüşüm sırasını kullanarak bir
% dönüşüm matrisi oluşturup, ardından bu matristen Axis-Angle'a dönüştüreceğiz.
% Simulink'teki VRML Viewer genellikle Z-Y-X konvansiyonunu iyi karşılar.

% Dönüşüm Matrisi Oluşturma (Z-Y-X Euler açısı sırası)
% R = Rz(psi) * Ry(theta) * Rx(phi)
Rx = [1 0 0; 0 cos(phi) -sin(phi); 0 sin(phi) cos(phi)];
Ry = [cos(theta) 0 sin(theta); 0 1 0; -sin(theta) 0 cos(theta)];
Rz = [cos(psi) -sin(psi) 0; sin(psi) cos(psi) 0; 0 0 1];

RotationMatrix = Rz * Ry * Rx;

% Dönüşüm Matrisinden Axis-Angle'a Dönüştürme
% (Bu dönüşüm için temel bir algoritma kullanılmıştır)
traceR = RotationMatrix(1,1) + RotationMatrix(2,2) + RotationMatrix(3,3);
angle = acos((traceR - 1) / 2);

if abs(angle) < 1e-6 % Açı çok küçükse veya sıfırsa
    axis = [0 0 1]; % Herhangi bir eksen olabilir, Z varsayalım
    angle = 0;
elseif abs(angle - pi) < 1e-6 % Açı 180 derece ise
    % Bu durum için daha dikkatli hesaplama gerekir,
    % örneğin sütunlar arası farklardan eksen bulunur.
    % Şimdilik bu durumu basitleştirelim veya varsayalım ki nadir olacak.
    % Daha sağlam bir yaklaşım için https://www.euclideanspace.com/maths/geometry/rotations/conversions/matrixToAngle/index.htm
    % gibi kaynaklara başvurulabilir.
    % Basit bir 180 derece dönüş ekseni bulma:
    axis_x = RotationMatrix(1,1) + 1;
    axis_y = RotationMatrix(2,2) + 1;
    axis_z = RotationMatrix(3,3) + 1;
    % En büyük bileşeni bulup normalize et
    max_val = max([axis_x, axis_y, axis_z]);
    if max_val == 0
        axis = [1 0 0]; % Varsayılan
    else
        axis = [axis_x, axis_y, axis_z] / max_val; % Normalizasyon sadece yönü korur.
    end
else
    % Normal durum
    axis_x = RotationMatrix(3,2) - RotationMatrix(2,3);
    axis_y = RotationMatrix(1,3) - RotationMatrix(3,1);
    axis_z = RotationMatrix(2,1) - RotationMatrix(1,2);
    axis_magnitude = norm([axis_x, axis_y, axis_z]);

    if axis_magnitude < 1e-6 % Neredeyse sıfır dönme
        axis = [0 0 1]; % Varsayılan
        angle = 0;
    else
        axis = [axis_x, axis_y, axis_z] / axis_magnitude;
    end
end

vrml_rot = [axis(1); axis(2); axis(3); angle];

end

== matlab function backstepping_last_good/spiral1 ==
  data: t input; ref_x output; ref_y output; ref_z output
function [ref_x, ref_y, ref_z] = fcn(t)
    % --- AYARLAR ---
    R = 15;          % Yarıçap (Sabit 5 metre)
    T_tur = 150;     % Bir tam turu kaç saniyede atsın?
    V_z = 0.5;      % Saniyede kaç metre yükselsin?
    
    % --- HESAPLAMA ---
    w = (2 * pi) / T_tur; % Açısal hız
    
    % Çember Denklemi (Sabit R ile)
    % t=0 anında (R, 0) noktasından başlar
    ref_x = R * cos(w * t); 
    ref_y = R * sin(w * t);
    
    % Yükseklik (Zamanla artar)
    ref_z = V_z * t;
end

== matlab function backstepping_last_good/sonsuzluk1 ==
  data: t input; ref_x output; ref_y output; ref_z output
function [ref_x, ref_y, ref_z] = fcn(t)
    % --- AYARLAR ---
    A = 50;          % Genişlik (X ekseni)
    B = 25;        % Yükseklik (Y ekseni)
    T_tur = 200;     % Sonsuzluk turu kaç saniyede atılsın?
    
    Hedef_Yukseklik = 15;   % Çıkılacak son irtifa (metre)
    T_yukselme = 20;        % 15 metreye kaç saniyede çıksın?
    
    % --- HESAPLAMA ---
    w = (2 * pi) / T_tur;
    
    % 1. X ve Y (Sonsuzluk Hareketi - 0,0'dan başlar)
    ref_x = A * sin(w * t);
    ref_y = B * sin(2 * w * t);
    
    % 2. Z (Yükselme Mantığı)
    % Eğer süre T_yukselme'den küçükse tırmanmaya devam et
    if t < T_yukselme
        % Doğrusal artış (Rampa)
        ref_z = (Hedef_Yukseklik / T_yukselme) * t;
    else
        % Hedefe ulaştıysa 15 metrede sabitle
        ref_z = Hedef_Yukseklik;
    end
    
end
